simulink model "MLP_networks"  (Simulink 7.7)
settings: Solver=ode45  StartTime=0.0  StopTime=10.0  RelTol=1e-3
libraries: neural x1629
(part 39 of 39)

== system MLP_networks/net_loc_rod_8_9/Layer 2/LW{2,1} ==
  "ad{2,1}" : Inport  PortDimensions=25
      mask Display: e = 0.06;c1 = [120 230 180]/255;c2 = ([120 230 180]+0)/(256+128);c3 = ([120 230 180]+128)/(256+128);patch([0 1 1 0],[0 0 1 1],c1);patch([0 1 1 1-e 1-e 0+e],[0 0 1 1-e 0+e 0+e],c2);patch([0 0 1 1-e 0+e 0+e],[0 1 1 1-e 1-e 0+e],c3);plot([0 1 1 0 0],[0 0 1 1 0]);
  "IW{2,1}(1,:)'" : Constant  Value=[-0.45447080635271114;-0.31431087999466095;0.23643842966814058;-0.26838264066697265;0.62158079059535698;0.64630925965078334;0.21776904252102494;0.92838649448024702;0.73391848601792298;-0.68443553978244875;-0.058262504733950955;-0.71107335585701004;-0.54591324791636819;0.31074562654655796;-0.94685307026245902;0.26887324589974526;0.010705518827699401;0.3796394579843112;0.34327649941262317;-1.1437670216094;0.90053987028130467;-0.10901199864440488;-1.1073873884529284;-0.86410791260520914;-0.92204914739905952]
      mask Display: e = 0.06;c1 = [120 150 230]/255;c2 = ([120 150 230]+0)/383;c3 = ([120 150 230]+128)/383;patch([0 1 1 0],[0 0 1 1],c1);patch([0 1 1 1-e 1-e 0+e],[0 0 1 1-e 0+e 0+e],c2);patch([0 0 1 1-e 0+e 0+e],[0 1 1 1-e 1-e 0+e],c3);plot([0 1 1 0 0],[0 0 1 1 0]);disp('weights');
  "IW{2,1}(10,:)'" : Constant  Value=[0.16261320114205341;0.85057219130381734;0.55243127341530673;-0.88195117415749713;-0.30049390446276986;-1.014955763686713;-0.41393637036512715;-0.93954442090004908;-0.56215105670641552;0.52952072507725989;0.85440080646791894;-0.00250141878530565;-0.2902870234308268;0.77038178692241177;1.0193322993447076;-0.29348678456992017;-0.45281217341190522;-0.45486860238087545;1.084604474121075;0.56344685224125202;-0.6458534409188561;0.86989576896543919;-0.67894851658584343;-0.072787712075929586;-0.088449026765616598]
      mask Display: e = 0.06;c1 = [120 150 230]/255;c2 = ([120 150 230]+0)/383;c3 = ([120 150 230]+128)/383;patch([0 1 1 0],[0 0 1 1],c1);patch([0 1 1 1-e 1-e 0+e],[0 0 1 1-e 0+e 0+e],c2);patch([0 0 1 1-e 0+e 0+e],[0 1 1 1-e 1-e 0+e],c3);plot([0 1 1 0 0],[0 0 1 1 0]);disp('weights');
  "IW{2,1}(11,:)'" : Constant  Value=[0.51216797701577244;-0.61438892099831866;1.2332181859604123;-1.2152438498115505;0.52251736025113349;-0.13914170551847893;-0.89663294252450099;0.1071591841447891;0.64626961438857278;-0.31974975626390789;0.90425624594228193;0.23311810869026173;0.57809497930447595;-0.51759015720995505;0.65776609000005626;-0.056587943103239377;1.0934578461807081;0.20012077737366696;0.38928601290892856;-0.069925753988291706;-0.46833581265105323;-0.56124207265295978;-0.89459244639724333;-0.70694327274206104;0.41313009557411701]
      mask Display: e = 0.06;c1 = [120 150 230]/255;c2 = ([120 150 230]+0)/383;c3 = ([120 150 230]+128)/383;patch([0 1 1 0],[0 0 1 1],c1);patch([0 1 1 1-e 1-e 0+e],[0 0 1 1-e 0+e 0+e],c2);patch([0 0 1 1-e 0+e 0+e],[0 1 1 1-e 1-e 0+e],c3);plot([0 1 1 0 0],[0 0 1 1 0]);disp('weights');
  "IW{2,1}(12,:)'" : Constant  Value=[-1.0367153164928766;-0.2086773626137968;-0.80832015596878137;0.1947198621022756;0.49348641081723604;0.044812146591478745;0.93317961128790405;-0.84837718445793697;-0.36841126818182129;-1.1224562126356763;-1.3423580142895108;-0.84409074802752404;-0.91276151182855159;-0.12584803107768913;-0.3402152433083459;-0.44504069889487502;-0.13012390121533071;0.46056376582825703;0.99075176834323464;0.095867520968736894;-0.58086488598308128;0.34331851844642508;1.0804134362946722;0.57636843085678846;0.0068501557111167151]
      mask Display: e = 0.06;c1 = [120 150 230]/255;c2 = ([120 150 230]+0)/383;c3 = ([120 150 230]+128)/383;patch([0 1 1 0],[0 0 1 1],c1);patch([0 1 1 1-e 1-e 0+e],[0 0 1 1-e 0+e 0+e],c2);patch([0 0 1 1-e 0+e 0+e],[0 1 1 1-e 1-e 0+e],c3);plot([0 1 1 0 0],[0 0 1 1 0]);disp('weights');
  "IW{2,1}(13,:)'" : Constant  Value=[-0.7243727430640643;-0.75325987047203258;0.32916868557887041;-0.87046233057132527;-0.40505034549515351;-0.73606709995248509;-0.57117708847133197;-0.028661557321403193;-0.12907256376571835;-0.70882230384049871;0.31678226521368041;-0.10082364388092978;0.6564749890771453;-0.049738012916444661;0.83422659334940041;-1.1296704058541949;0.94089271777742445;0.15949922140755984;-0.10705922974869457;0.87697187766797047;-1.0866913744390712;-0.71353658871453851;-0.31873702515843627;-0.252881252085425;-1.0189008728429951]
      mask Display: e = 0.06;c1 = [120 150 230]/255;c2 = ([120 150 230]+0)/383;c3 = ([120 150 230]+128)/383;patch([0 1 1 0],[0 0 1 1],c1);patch([0 1 1 1-e 1-e 0+e],[0 0 1 1-e 0+e 0+e],c2);patch([0 0 1 1-e 0+e 0+e],[0 1 1 1-e 1-e 0+e],c3);plot([0 1 1 0 0],[0 0 1 1 0]);disp('weights');
  "IW{2,1}(14,:)'" : Constant  Value=[0.53371665285306602;-0.76095279927957649;-0.094308089491326283;0.80974430444344658;-1.0601529091744661;-0.57891757482366835;0.032455299426623785;-0.37525233439382483;-0.8579469021295838;0.83494699788668525;0.049205853924271216;-0.77709270533384189;0.19868335805748968;-0.88504930806369408;-0.095340804143279015;0.52800234434791515;-0.43233621624610419;-0.64289579789318352;0.75364398055159043;0.77792715087691144;0.63464043036909801;-0.21444243504652935;0.52064758843423997;-0.90369622137036576;-0.93600425626526274]
      mask Display: e = 0.06;c1 = [120 150 230]/255;c2 = ([120 150 230]+0)/383;c3 = ([120 150 230]+128)/383;patch([0 1 1 0],[0 0 1 1],c1);patch([0 1 1 1-e 1-e 0+e],[0 0 1 1-e 0+e 0+e],c2);patch([0 0 1 1-e 0+e 0+e],[0 1 1 1-e 1-e 0+e],c3);plot([0 1 1 0 0],[0 0 1 1 0]);disp('weights');
  "IW{2,1}(15,:)'" : Constant  Value=[0.37541716291702742;-0.21193619710435674;-0.94576323987022948;0.34691220420858604;-0.38907419761502582;0.84729396197252627;0.61247771158965003;1.0019605765670976;-0.045197648782573069;-1.1799168746424504;0.84852837950369564;-0.81099574040787803;0.1941658430896363;-0.010229454310141418;0.44591624310136047;-0.38010130538266051;-0.75205589528395445;0.60044481822345563;0.82055369407816969;0.053523240861982138;1.2391033690142557;-0.54989802212004923;-0.14511814137346626;-0.33145647268207051;0.56500446191282006]
      mask Display: e = 0.06;c1 = [120 150 230]/255;c2 = ([120 150 230]+0)/383;c3 = ([120 150 230]+128)/383;patch([0 1 1 0],[0 0 1 1],c1);patch([0 1 1 1-e 1-e 0+e],[0 0 1 1-e 0+e 0+e],c2);patch([0 0 1 1-e 0+e 0+e],[0 1 1 1-e 1-e 0+e],c3);plot([0 1 1 0 0],[0 0 1 1 0]);disp('weights');
  "IW{2,1}(16,:)'" : Constant  Value=[-1.0394652666780868;0.15085289490948153;0.44339428350864968;-0.77309686754184659;-0.33808340538731163;-1.1935669085568268;-0.63097259795222405;0.299249348653851;0.92160773792947315;-1.0044893892944822;0.40875287808051819;-0.12022115639313204;-0.4889679626946678;1.0578373529209588;0.6070540991902259;0.9876432388180314;0.32942173306276984;0.08451986358521997;-0.1855524467079297;0.70927078909658214;0.77583003077482993;-0.087847247331581058;0.58774596387649525;-0.62544316719270998;-0.35284088943191494]
      mask Display: e = 0.06;c1 = [120 150 230]/255;c2 = ([120 150 230]+0)/383;c3 = ([120 150 230]+128)/383;patch([0 1 1 0],[0 0 1 1],c1);patch([0 1 1 1-e 1-e 0+e],[0 0 1 1-e 0+e 0+e],c2);patch([0 0 1 1-e 0+e 0+e],[0 1 1 1-e 1-e 0+e],c3);plot([0 1 1 0 0],[0 0 1 1 0]);disp('weights');
  "IW{2,1}(17,:)'" : Constant  Value=[0.34126724354609184;0.73618068075490573;0.61771615039297245;-0.75619007627092016;0.098089840878866116;-0.966566899104913;0.5073556368631954;1.027292936105652;0.21560095819971478;-0.2639067977294588;-0.710128333782023;-0.35468195912204459;0.62972345593633328;0.088918966245724623;-0.57676352850483459;0.59235109654670703;0.62310731853968448;1.0120009144022506;0.28344383729740075;-0.67135974215603889;0.53291075314000347;0.92992562657934774;0.045942961126403739;-0.97360891231881208;-0.8952773597675806]
      mask Display: e = 0.06;c1 = [120 150 230]/255;c2 = ([120 150 230]+0)/383;c3 = ([120 150 230]+128)/383;patch([0 1 1 0],[0 0 1 1],c1);patch([0 1 1 1-e 1-e 0+e],[0 0 1 1-e 0+e 0+e],c2);patch([0 0 1 1-e 0+e 0+e],[0 1 1 1-e 1-e 0+e],c3);plot([0 1 1 0 0],[0 0 1 1 0]);disp('weights');
  "IW{2,1}(18,:)'" : Constant  Value=[-0.098397319648461698;-1.1310897911939402;0.20417535507397502;-0.7539013471598266;0.68442491292076157;0.25093656866891895;-1.1397774937477676;0.12159248155228496;0.7780135310512547;0.035538843403749382;-0.91235298915348495;-1.0000341549927907;0.79208580035862641;0.00074876713405867118;-0.31150935626008885;-0.96556344356727131;-0.4361193934911502;0.1376261764682912;0.59882639597992626;-0.42398383503226761;1.1604296296421897;-0.21284418619408138;0.34961610435553286;0.084401125103079372;-0.72242990170213894]
      mask Display: e = 0.06;c1 = [120 150 230]/255;c2 = ([120 150 230]+0)/383;c3 = ([120 150 230]+128)/383;patch([0 1 1 0],[0 0 1 1],c1);patch([0 1 1 1-e 1-e 0+e],[0 0 1 1-e 0+e 0+e],c2);patch([0 0 1 1-e 0+e 0+e],[0 1 1 1-e 1-e 0+e],c3);plot([0 1 1 0 0],[0 0 1 1 0]);disp('weights');
  "IW{2,1}(19,:)'" : Constant  Value=[0.78773378785982129;-0.48036277769725011;-0.47045729207981185;-1.0285380769624823;0.57946471346881834;-1.0274103528129928;-0.48201049424572456;0.33639731381638377;0.83791439406269541;-0.74451317574282194;-0.51790206635491542;0.25105315003569045;0.48285725406315255;0.81142022830880567;-0.93247588992234043;-0.62647816753072572;0.15040280733987643;0.65792099584298835;0.37927369980568609;-0.81003399537479481;-0.62849242597305155;0.068466355370222956;-0.30458643155508885;0.08181346905433419;-0.87104728264235998]
      mask Display: e = 0.06;c1 = [120 150 230]/255;c2 = ([120 150 230]+0)/383;c3 = ([120 150 230]+128)/383;patch([0 1 1 0],[0 0 1 1],c1);patch([0 1 1 1-e 1-e 0+e],[0 0 1 1-e 0+e 0+e],c2);patch([0 0 1 1-e 0+e 0+e],[0 1 1 1-e 1-e 0+e],c3);plot([0 1 1 0 0],[0 0 1 1 0]);disp('weights');
  "IW{2,1}(2,:)'" : Constant  Value=[0.96230663942317574;-0.44935662887228023;-0.56623021211938263;-0.98970111008255923;-0.17258463946061253;-0.86731106367562238;0.74381718631924409;0.6694547609833591;0.75417674683607538;-1.0130175782751791;0.99952362222759994;0.37793136884111361;-0.5244440690711103;-0.34430315584704518;-0.78883180270087583;0.74499763515124462;0.34936053745594026;-0.28074185014234565;-0.59199610119552726;0.28196716663522736;0.95011394088102452;-0.69131758403450982;-0.05622148048795448;-0.85996969469457929;0.28393870377919894]
      mask Display: e = 0.06;c1 = [120 150 230]/255;c2 = ([120 150 230]+0)/383;c3 = ([120 150 230]+128)/383;patch([0 1 1 0],[0 0 1 1],c1);patch([0 1 1 1-e 1-e 0+e],[0 0 1 1-e 0+e 0+e],c2);patch([0 0 1 1-e 0+e 0+e],[0 1 1 1-e 1-e 0+e],c3);plot([0 1 1 0 0],[0 0 1 1 0]);disp('weights');
  "IW{2,1}(20,:)'" : Constant  Value=[0.86417986057223173;-0.71409214147296729;0.87649163618636761;-0.26966100345125088;0.22235648369379468;0.58221344515541951;0.49784067504208446;0.97207961406944532;0.9071543515886572;0.68777222135818183;-0.042949087236494599;0.59168218732534095;-0.12077111467202464;0.79259172488769247;-0.45576896748524726;-0.50437719394637759;-0.70249062368748016;0.89245706256996071;0.88961506239928179;0.72849965232042246;-0.026521615511835725;0.079500787307071025;-0.43713934870209875;-0.80163782346974666;-0.83869567670330147]
      mask Display: e = 0.06;c1 = [120 150 230]/255;c2 = ([120 150 230]+0)/383;c3 = ([120 150 230]+128)/383;patch([0 1 1 0],[0 0 1 1],c1);patch([0 1 1 1-e 1-e 0+e],[0 0 1 1-e 0+e 0+e],c2);patch([0 0 1 1-e 0+e 0+e],[0 1 1 1-e 1-e 0+e],c3);plot([0 1 1 0 0],[0 0 1 1 0]);disp('weights');
  "IW{2,1}(21,:)'" : Constant  Value=[0.1911532386158688;0.1621449493425382;-0.93637196968629799;-0.26400809382302576;0.54569865597064104;0.88748772662652009;0.50077218719541849;0.67412697249317532;0.40883495027129241;-0.092833189717247674;-0.74794325847843501;-0.60048439500264339;0.40310127003620538;-0.28964783835670249;-0.94317412015928992;0.85095667464863523;-0.17069104715442765;0.58499249929003749;-1.0048085585643964;0.23236160394851982;-0.48000714163089853;-1.000876063264845;0.99191080162000533;0.80503319313583599;-0.51157270112970599]
      mask Display: e = 0.06;c1 = [120 150 230]/255;c2 = ([120 150 230]+0)/383;c3 = ([120 150 230]+128)/383;patch([0 1 1 0],[0 0 1 1],c1);patch([0 1 1 1-e 1-e 0+e],[0 0 1 1-e 0+e 0+e],c2);patch([0 0 1 1-e 0+e 0+e],[0 1 1 1-e 1-e 0+e],c3);plot([0 1 1 0 0],[0 0 1 1 0]);disp('weights');
  "IW{2,1}(22,:)'" : Constant  Value=[0.9320611787902402;0.28364314918527139;-0.20093614072570032;-0.3751052916383622;-0.52578913527537752;0.70237214101441625;-1.0319590808387713;-0.85558263819382308;0.88270969846196012;-0.46751281861565375;-0.91417776486314584;0.31547930902410298;0.81163899116420279;-0.15828942492757292;-0.24707285170931548;-0.39170449380734118;-0.88386960061365805;1.1541453664581989;0.78038688405888279;0.5306796455286874;0.34440910112714629;-0.33799086462182248;0.8850373797599308;-0.63028138227995167;0.17673160463486462]
      mask Display: e = 0.06;c1 = [120 150 230]/255;c2 = ([120 150 230]+0)/383;c3 = ([120 150 230]+128)/383;patch([0 1 1 0],[0 0 1 1],c1);patch([0 1 1 1-e 1-e 0+e],[0 0 1 1-e 0+e 0+e],c2);patch([0 0 1 1-e 0+e 0+e],[0 1 1 1-e 1-e 0+e],c3);plot([0 1 1 0 0],[0 0 1 1 0]);disp('weights');
  "IW{2,1}(23,:)'" : Constant  Value=[-0.82185203974927235;0.92891702155408973;-0.37877676349477202;-0.62190517768300357;0.32818732774692172;0.0038303412033409774;-0.14571980217775737;0.80249850052066751;-0.63021858125598862;0.78492448828022865;-0.94038973664783887;0.71945342383225364;-0.93285472625417609;-0.32614841235081482;0.73697057015097023;-0.38846684548949634;0.88920720011482535;0.20290850509137778;-0.84560863661300678;-0.16868606751307699;-0.84819165523872442;-0.40115615282001765;-0.65920959088980569;0.72810794552070213;-0.25217760313611665]
      mask Display: e = 0.06;c1 = [120 150 230]/255;c2 = ([120 150 230]+0)/383;c3 = ([120 150 230]+128)/383;patch([0 1 1 0],[0 0 1 1],c1);patch([0 1 1 1-e 1-e 0+e],[0 0 1 1-e 0+e 0+e],c2);patch([0 0 1 1-e 0+e 0+e],[0 1 1 1-e 1-e 0+e],c3);plot([0 1 1 0 0],[0 0 1 1 0]);disp('weights');
  "IW{2,1}(24,:)'" : Constant  Value=[0.30582931147396802;-0.036178013157462559;-0.55531656899262816;0.76280973892360027;-0.03762136036114589;-0.76339575584342301;0.99723793513686021;-0.48053176437438622;0.7936960673034823;-0.47389009352160244;-0.12021842780939135;-1.0176735468094926;1.0051963883138231;0.53389548534064435;0.62406304753365782;-0.45167165089064937;-0.18484523206284098;-0.88667933177244607;0.59183228168738489;-0.71299173383454761;0.59431335267309748;-0.83985050387188986;0.59717562904826715;0.75949420856795158;0.39693109681614497]
      mask Display: e = 0.06;c1 = [120 150 230]/255;c2 = ([120 150 230]+0)/383;c3 = ([120 150 230]+128)/383;patch([0 1 1 0],[0 0 1 1],c1);patch([0 1 1 1-e 1-e 0+e],[0 0 1 1-e 0+e 0+e],c2);patch([0 0 1 1-e 0+e 0+e],[0 1 1 1-e 1-e 0+e],c3);plot([0 1 1 0 0],[0 0 1 1 0]);disp('weights');
  "IW{2,1}(25,:)'" : Constant  Value=[-1.0684009758474187;1.1722115613612545;-0.57111187175963052;-0.8878679369744843;1.1295127330090828;0.44904490314857132;0.14031476727547645;0.08735425437740639;-0.34565747025485005;-0.72178721361568943;0.59197326673989126;-0.42068869129676106;-0.82095323234120809;-0.82414047258516032;0.056752643726297583;-0.0579096547071552;0.271312447793641;0.89147339407483417;0.17874804668826502;-0.10936602263727534;0.3520689038399139;-0.76695586884888844;-0.43345975693307037;0.88579403742493612;0.47182323470607712]
      mask Display: e = 0.06;c1 = [120 150 230]/255;c2 = ([120 150 230]+0)/383;c3 = ([120 150 230]+128)/383;patch([0 1 1 0],[0 0 1 1],c1);patch([0 1 1 1-e 1-e 0+e],[0 0 1 1-e 0+e 0+e],c2);patch([0 0 1 1-e 0+e 0+e],[0 1 1 1-e 1-e 0+e],c3);plot([0 1 1 0 0],[0 0 1 1 0]);disp('weights');
  "IW{2,1}(26,:)'" : Constant  Value=[0.77450591200359475;0.91270531388688547;0.83574788691334789;-0.34502986728419421;-0.55790971192747163;-0.72070283837337334;0.20504475257688248;-0.83640939284270199;0.64277075785744209;-0.57192213445216011;0.32327000181573323;-0.68416799747796198;-0.90528107143746939;-0.10217138652846579;0.73971597769657271;0.89218725128765564;0.29840745150663905;-0.5450647450867212;-0.73235030444179139;-0.58115961231792035;0.63460766784378642;0.40333367981231855;-0.89475280670748758;0.65293566293097571;0.12099389597776294]
      mask Display: e = 0.06;c1 = [120 150 230]/255;c2 = ([120 150 230]+0)/383;c3 = ([120 150 230]+128)/383;patch([0 1 1 0],[0 0 1 1],c1);patch([0 1 1 1-e 1-e 0+e],[0 0 1 1-e 0+e 0+e],c2);patch([0 0 1 1-e 0+e 0+e],[0 1 1 1-e 1-e 0+e],c3);plot([0 1 1 0 0],[0 0 1 1 0]);disp('weights');
  "IW{2,1}(27,:)'" : Constant  Value=[0.61217593788432589;1.0105744665838057;0.10860586955594799;0.94251107889473051;-0.88010468086265536;1.0106862859418371;0.97539560690599569;0.50827419220215719;0.59801040058874899;-0.039371834639818012;0.42615970864737573;0.40800828356563923;0.5757827372943547;0.85016099941120338;0.89746531145472463;0.080547975206119823;0.090172289218227619;-0.87795208623074783;0.69526781873484145;-0.45630044385637419;-0.17710867995277463;0.76421683404438578;-0.41404996922286047;-0.32332715019168495;-0.36597634722835087]
      mask Display: e = 0.06;c1 = [120 150 230]/255;c2 = ([120 150 230]+0)/383;c3 = ([120 150 230]+128)/383;patch([0 1 1 0],[0 0 1 1],c1);patch([0 1 1 1-e 1-e 0+e],[0 0 1 1-e 0+e 0+e],c2);patch([0 0 1 1-e 0+e 0+e],[0 1 1 1-e 1-e 0+e],c3);plot([0 1 1 0 0],[0 0 1 1 0]);disp('weights');
  "IW{2,1}(28,:)'" : Constant  Value=[-0.92362832193853739;0.29233412368150907;-0.28036118684992595;-0.52775115853329257;1.1089509079989204;0.17905600152632489;0.46663393694438871;-0.37191504490185906;-0.17999421651757258;0.058306317753163014;-1.0140410146243994;-0.11183420954904957;0.98413115720863986;0.16517689889845533;0.88854308219033906;-1.0667065996248886;0.60226014665316829;-0.96893529625524433;-0.5008750006416941;0.022413819844856471;-0.62628687438953801;0.42127137893488054;0.15159245687022385;1.0789682742542015;0.56723459454054859]
      mask Display: e = 0.06;c1 = [120 150 230]/255;c2 = ([120 150 230]+0)/383;c3 = ([120 150 230]+128)/383;patch([0 1 1 0],[0 0 1 1],c1);patch([0 1 1 1-e 1-e 0+e],[0 0 1 1-e 0+e 0+e],c2);patch([0 0 1 1-e 0+e 0+e],[0 1 1 1-e 1-e 0+e],c3);plot([0 1 1 0 0],[0 0 1 1 0]);disp('weights');
  "IW{2,1}(29,:)'" : Constant  Value=[-0.75071122167525839;-0.16377370234095223;1.0432309786139491;-0.9419284667685428;0.76379982457742834;0.43959955342497242;-0.76278982989123456;0.10257817545510309;0.74004434461333557;0.83753673819670804;0.13167611675610816;0.76014534213608953;-0.66457009872673756;0.36592785804355776;-0.6120363225355574;-0.488276829481398;-0.6618208484555782;-0.11194073805334005;0.22043830882817622;-0.40349829775212342;0.47209337717495281;-0.87514000467748676;-0.74737020827019207;-0.96943693375218565;0.64256521052270565]
      mask Display: e = 0.06;c1 = [120 150 230]/255;c2 = ([120 150 230]+0)/383;c3 = ([120 150 230]+128)/383;patch([0 1 1 0],[0 0 1 1],c1);patch([0 1 1 1-e 1-e 0+e],[0 0 1 1-e 0+e 0+e],c2);patch([0 0 1 1-e 0+e 0+e],[0 1 1 1-e 1-e 0+e],c3);plot([0 1 1 0 0],[0 0 1 1 0]);disp('weights');
  "IW{2,1}(3,:)'" : Constant  Value=[-0.72661874690638639;0.98304485670167907;-0.39280364502085141;0.30668407085875982;-0.230114863701743;0.43303809144138394;0.7277239726221405;0.99977015994841312;0.87853696172551077;0.1970889781751029;-0.97320525276089309;0.56460947642782677;0.32677707421560953;-0.32048198505949954;0.50614504721549824;-0.45383421909495375;0.92994931318815421;-0.39720128292223061;0.92109540405251633;-0.71483440373770279;0.85524274992117122;-0.069813992173348174;-0.5834831065067082;0.81005318020036188;0.33671550153450908]
      mask Display: e = 0.06;c1 = [120 150 230]/255;c2 = ([120 150 230]+0)/383;c3 = ([120 150 230]+128)/383;patch([0 1 1 0],[0 0 1 1],c1);patch([0 1 1 1-e 1-e 0+e],[0 0 1 1-e 0+e 0+e],c2);patch([0 0 1 1-e 0+e 0+e],[0 1 1 1-e 1-e 0+e],c3);plot([0 1 1 0 0],[0 0 1 1 0]);disp('weights');
  "IW{2,1}(30,:)'" : Constant  Value=[0.9520365997944269;0.5784099977345214;0.74134421413668339;-0.06363803828697058;-1.0124114735802598;-0.093182754887791014;-0.20269235928731327;-0.094131170798026784;0.80239368351042095;0.27621364652589353;-0.39945726685966931;0.38509994188586416;0.76957868255844897;-0.55737306059620473;0.88795019251236396;1.2044289516558007;0.13452228364405522;0.51460777295093929;0.3092540981712541;-0.68222047984635237;0.01906913268519532;-0.37617379142855234;0.93628982587397003;-1.0441754001006984;0.068380270421470518]
      mask Display: e = 0.06;c1 = [120 150 230]/255;c2 = ([120 150 230]+0)/383;c3 = ([120 150 230]+128)/383;patch([0 1 1 0],[0 0 1 1],c1);patch([0 1 1 1-e 1-e 0+e],[0 0 1 1-e 0+e 0+e],c2);patch([0 0 1 1-e 0+e 0+e],[0 1 1 1-e 1-e 0+e],c3);plot([0 1 1 0 0],[0 0 1 1 0]);disp('weights');
  "IW{2,1}(31,:)'" : Constant  Value=[0.15567714868126017;-0.072085627004655969;-0.050397630838470736;0.95833156808844622;-0.1879410696794612;-0.59649025386386878;0.84553357656875139;0.61551922306369911;-0.9713825097799843;0.4979667076348453;0.26631163648564493;-0.17892940121863304;-0.051055201034569529;-1.1033606312967341;-0.18636221888045618;1.2140195934896645;-0.43500698384749537;-0.51998517385757448;-1.1353997625882177;0.85700759160672535;0.47407089976182043;-0.51827476400697037;0.06559682343247443;-0.911672680644522;-0.15377455532303921]
      mask Display: e = 0.06;c1 = [120 150 230]/255;c2 = ([120 150 230]+0)/383;c3 = ([120 150 230]+128)/383;patch([0 1 1 0],[0 0 1 1],c1);patch([0 1 1 1-e 1-e 0+e],[0 0 1 1-e 0+e 0+e],c2);patch([0 0 1 1-e 0+e 0+e],[0 1 1 1-e 1-e 0+e],c3);plot([0 1 1 0 0],[0 0 1 1 0]);disp('weights');
  "IW{2,1}(32,:)'" : Constant  Value=[0.82909455037823787;0.99714319599564616;1.1139332023334763;0.54654892769062013;0.52131269431691585;-0.80449944267326734;0.55664826096035924;-1.002741723350306;-0.01985018005497385;-0.67254734982516517;-0.93662079473490822;-0.03014214992894999;1.0464148662521608;0.15910202671912124;1.2862964972491364;0.45764157957773155;0.71356320912522109;-0.42510632495263323;-0.69440295242741623;-0.0045543062036582822;0.035464232309733092;-0.19904714832607096;0.1444002491346317;0.040868735796712262;0.083526646292963455]
      mask Display: e = 0.06;c1 = [120 150 230]/255;c2 = ([120 150 230]+0)/383;c3 = ([120 150 230]+128)/383;patch([0 1 1 0],[0 0 1 1],c1);patch([0 1 1 1-e 1-e 0+e],[0 0 1 1-e 0+e 0+e],c2);patch([0 0 1 1-e 0+e 0+e],[0 1 1 1-e 1-e 0+e],c3);plot([0 1 1 0 0],[0 0 1 1 0]);disp('weights');
  "IW{2,1}(33,:)'" : Constant  Value=[0.036631572386991482;-0.4859312403210907;0.47210982987621547;0.89311539401184092;0.62724039374736873;-0.75762622064522089;-0.22116005207619702;-1.0000476620174505;0.88242383389663503;0.87406908733565825;0.27178801741200337;-0.85961354623926522;0.80446421087919417;0.94536513407364309;0.67862529152930817;-0.11239854292815231;0.48071669928340838;-0.21685603275548129;-0.018082263103240091;-1.0018384755236334;-0.74941988688188865;0.14514850868224274;0.19341587119424772;-0.95315483233896936;0.087088605244087264]
      mask Display: e = 0.06;c1 = [120 150 230]/255;c2 = ([120 150 230]+0)/383;c3 = ([120 150 230]+128)/383;patch([0 1 1 0],[0 0 1 1],c1);patch([0 1 1 1-e 1-e 0+e],[0 0 1 1-e 0+e 0+e],c2);patch([0 0 1 1-e 0+e 0+e],[0 1 1 1-e 1-e 0+e],c3);plot([0 1 1 0 0],[0 0 1 1 0]);disp('weights');
  "IW{2,1}(34,:)'" : Constant  Value=[0.53373781853001401;1.0854542172297528;-0.050268462275507235;0.18814361980720323;-0.19858976628212019;0.95097137761216377;-1.0046101954080138;-0.16748350752219901;-0.072886125187907491;-0.95017139866892542;-0.7534524616942313;-1.0120494484012044;-0.30821221046317987;0.3623711234025066;-0.032567929132316251;-1.1176982715758284;0.19097961349793782;0.37497120131263378;0.69756716041654054;0.97114030711281907;-0.99072273810272415;0.32529142645115866;0.5459282808151813;-0.46238529402502659;0.31491921013096502]
      mask Display: e = 0.06;c1 = [120 150 230]/255;c2 = ([120 150 230]+0)/383;c3 = ([120 150 230]+128)/383;patch([0 1 1 0],[0 0 1 1],c1);patch([0 1 1 1-e 1-e 0+e],[0 0 1 1-e 0+e 0+e],c2);patch([0 0 1 1-e 0+e 0+e],[0 1 1 1-e 1-e 0+e],c3);plot([0 1 1 0 0],[0 0 1 1 0]);disp('weights');
  "IW{2,1}(35,:)'" : Constant  Value=[0.51979428844107578;0.80936660991970011;0.89434175320810017;0.22804712757419968;-0.39797463477756434;-0.16323079404302634;-0.28184633595783565;-0.80960057310033162;-0.91452441576709198;-0.70296872148801859;0.34996440277301383;0.60428302086858032;-0.33764774632615158;-0.9516367577091448;0.17289559134218208;1.0099555310096149;0.65922170646939704;-0.90277879989919618;0.61983937615839846;-0.93840826454856285;-0.50370480019087227;-0.47833541448699218;-0.85582425731092604;0.37359779335281229;-0.60469184067102733]
      mask Display: e = 0.06;c1 = [120 150 230]/255;c2 = ([120 150 230]+0)/383;c3 = ([120 150 230]+128)/383;patch([0 1 1 0],[0 0 1 1],c1);patch([0 1 1 1-e 1-e 0+e],[0 0 1 1-e 0+e 0+e],c2);patch([0 0 1 1-e 0+e 0+e],[0 1 1 1-e 1-e 0+e],c3);plot([0 1 1 0 0],[0 0 1 1 0]);disp('weights');
  "IW{2,1}(36,:)'" : Constant  Value=[-0.23384974203236852;-0.54113992244807474;1.1016650872942653;1.1867094141570538;-0.18259887724139948;-0.61650306840294833;-1.0579748981135972;-0.86695949316505472;0.34258323344695207;0.25134154100917466;0.49668598978421058;1.0874547853160808;0.33877522986499109;0.07278981615384239;-0.93246428697756634;-0.49415699510248245;-0.61347936617450993;0.96312184078209462;-0.31995152917786074;-0.49914549720953977;0.26822355945592924;-0.66445453280374978;0.065126988778028916;-0.74467649600230734;0.31341549290898102]
      mask Display: e = 0.06;c1 = [120 150 230]/255;c2 = ([120 150 230]+0)/383;c3 = ([120 150 230]+128)/383;patch([0 1 1 0],[0 0 1 1],c1);patch([0 1 1 1-e 1-e 0+e],[0 0 1 1-e 0+e 0+e],c2);patch([0 0 1 1-e 0+e 0+e],[0 1 1 1-e 1-e 0+e],c3);plot([0 1 1 0 0],[0 0 1 1 0]);disp('weights');
  "IW{2,1}(37,:)'" : Constant  Value=[0.62394894755522512;-0.72463106030111668;-0.28915310904051367;0.38031615254904;0.96336050725290678;0.94026979907725095;0.45200410654678858;0.77127112338602177;-0.42381660866722354;-1.0203299574836318;0.055877914679506882;-0.46593533880670451;0.91323202709270723;-0.86505688276390513;0.021478310200374332;0.9544367752917674;-0.70347566787313309;-0.54726505052392349;-0.56606452403588858;0.78215767993104612;0.40928629022026891;0.078962355906479584;-0.84847545453080819;0.16386319596577098;-0.48167518437484919]
      mask Display: e = 0.06;c1 = [120 150 230]/255;c2 = ([120 150 230]+0)/383;c3 = ([120 150 230]+128)/383;patch([0 1 1 0],[0 0 1 1],c1);patch([0 1 1 1-e 1-e 0+e],[0 0 1 1-e 0+e 0+e],c2);patch([0 0 1 1-e 0+e 0+e],[0 1 1 1-e 1-e 0+e],c3);plot([0 1 1 0 0],[0 0 1 1 0]);disp('weights');
  "IW{2,1}(38,:)'" : Constant  Value=[-0.82263192954369435;0.37012724951292331;0.74972080760741266;1.0351005528830399;0.56512505853040529;-0.81539680330377129;0.39072051088000676;-0.29041608151021198;-0.0087149107531334213;0.74173699894930678;0.11484230430867111;0.87839370487535939;0.2494334766034727;0.11682233387751935;0.69415268384814743;-0.04027180420643884;-0.11770698203286697;-0.1421206021269576;0.67417577094500547;-0.75587535966966957;-1.1957762438779307;0.89939892311584302;-0.77485709288092064;0.10804837880923522;1.1712256256702318]
      mask Display: e = 0.06;c1 = [120 150 230]/255;c2 = ([120 150 230]+0)/383;c3 = ([120 150 230]+128)/383;patch([0 1 1 0],[0 0 1 1],c1);patch([0 1 1 1-e 1-e 0+e],[0 0 1 1-e 0+e 0+e],c2);patch([0 0 1 1-e 0+e 0+e],[0 1 1 1-e 1-e 0+e],c3);plot([0 1 1 0 0],[0 0 1 1 0]);disp('weights');
  "IW{2,1}(39,:)'" : Constant  Value=[-0.087941008322375919;-1.2617558070192225;0.81267471888099152;-0.095310299855226308;-0.14430690024522641;-0.59215209219935194;-0.24621944251458036;1.0141764718422999;-0.72126979904741317;-0.24786972627093884;-0.85079063426578938;-0.2060494957307637;0.17468343830161173;-0.20772011445927371;0.83117698885287106;-0.8259244632319398;-0.72584811323123788;-0.50446335809251608;0.30702358162880289;-0.22927699911977933;0.7303610645550993;-0.67473178861566885;0.565406694916473;0.0085444645835071244;1.2613327692520118]
      mask Display: e = 0.06;c1 = [120 150 230]/255;c2 = ([120 150 230]+0)/383;c3 = ([120 150 230]+128)/383;patch([0 1 1 0],[0 0 1 1],c1);patch([0 1 1 1-e 1-e 0+e],[0 0 1 1-e 0+e 0+e],c2);patch([0 0 1 1-e 0+e 0+e],[0 1 1 1-e 1-e 0+e],c3);plot([0 1 1 0 0],[0 0 1 1 0]);disp('weights');
  "IW{2,1}(4,:)'" : Constant  Value=[-0.91763924018682308;-0.14482416183886465;-0.81975295697163553;0.50338071021686293;1.1036741771908423;0.31005456238123802;0.86665074311709989;0.30585124448433609;0.051290156212662578;-0.6974987566200439;0.18478498207816629;0.47363312320663153;-0.073589393868213546;-1.045358662826845;0.82981806326454777;0.95650149909522542;-0.37939447955152711;0.43646379385359629;0.076893257963874376;0.89801851174081115;1.0491188749862304;0.36373872441237598;0.37760536648727727;-0.47948700442506348;0.70507282134646909]
      mask Display: e = 0.06;c1 = [120 150 230]/255;c2 = ([120 150 230]+0)/383;c3 = ([120 150 230]+128)/383;patch([0 1 1 0],[0 0 1 1],c1);patch([0 1 1 1-e 1-e 0+e],[0 0 1 1-e 0+e 0+e],c2);patch([0 0 1 1-e 0+e 0+e],[0 1 1 1-e 1-e 0+e],c3);plot([0 1 1 0 0],[0 0 1 1 0]);disp('weights');
  "IW{2,1}(40,:)'" : Constant  Value=[0.10117395120403073;0.24715881593069883;0.83728045669710482;-0.18671601343198624;0.069509096529898423;-0.19742449946957311;0.83344649776616908;1.3106956705379531;-0.2462286395319955;-0.90486362677857146;0.54701955067878771;0.89670157241501358;0.35229560876483135;0.66802678717329667;0.063332974454404695;-0.46645975844027782;1.3814570160061039;-0.33411412115441702;-0.42341112280074589;-0.62588934616862224;-1.2228788212487895;-0.44646354140142547;0.23884228407282401;-0.9311058974493388;0.78530320127861797]
      mask Display: e = 0.06;c1 = [120 150 230]/255;c2 = ([120 150 230]+0)/383;c3 = ([120 150 230]+128)/383;patch([0 1 1 0],[0 0 1 1],c1);patch([0 1 1 1-e 1-e 0+e],[0 0 1 1-e 0+e 0+e],c2);patch([0 0 1 1-e 0+e 0+e],[0 1 1 1-e 1-e 0+e],c3);plot([0 1 1 0 0],[0 0 1 1 0]);disp('weights');
  "IW{2,1}(5,:)'" : Constant  Value=[1.0939965012744106;-0.66742083860121626;0.44176116557230544;0.19488103679144;-0.41864394361289581;-0.97783478160897297;-0.24004993526630705;-0.71760852479943238;0.65681332424103389;-0.21988704460819664;-0.5813359133985625;-0.34065285262784456;0.9033686873923521;-0.62892988549260465;0.88227040548382951;-0.98957493871181734;-0.18279002704064404;0.81324318493551628;-0.5523906417857144;0.64071395311200929;-0.44341231540924431;-0.70364701527976248;-0.55889331586038327;0.57611249338715798;-0.80142859703937419]
      mask Display: e = 0.06;c1 = [120 150 230]/255;c2 = ([120 150 230]+0)/383;c3 = ([120 150 230]+128)/383;patch([0 1 1 0],[0 0 1 1],c1);patch([0 1 1 1-e 1-e 0+e],[0 0 1 1-e 0+e 0+e],c2);patch([0 0 1 1-e 0+e 0+e],[0 1 1 1-e 1-e 0+e],c3);plot([0 1 1 0 0],[0 0 1 1 0]);disp('weights');
  "IW{2,1}(6,:)'" : Constant  Value=[0.52672972175919663;-0.54234069679748398;0.26229992785495393;-0.43950033724518695;-0.47671006602958749;-0.4084766690695722;-0.36069666513241849;0.96896850921895872;1.0365754228866313;0.016908975229810146;-0.48417792757850503;0.78272104705523271;-0.053406657320566486;0.41691219365676491;-0.50300491903087408;-1.2337188253843483;0.94909946627070729;-0.44246513377777069;-0.66330401220892377;-0.0034619098097734263;0.5949373079918362;0.48162040059480948;1.0523240380352006;0.89633573238191411;-0.36727415959127846]
      mask Display: e = 0.06;c1 = [120 150 230]/255;c2 = ([120 150 230]+0)/383;c3 = ([120 150 230]+128)/383;patch([0 1 1 0],[0 0 1 1],c1);patch([0 1 1 1-e 1-e 0+e],[0 0 1 1-e 0+e 0+e],c2);patch([0 0 1 1-e 0+e 0+e],[0 1 1 1-e 1-e 0+e],c3);plot([0 1 1 0 0],[0 0 1 1 0]);disp('weights');
  "IW{2,1}(7,:)'" : Constant  Value=[-0.92097304747775321;0.77184685775303008;0.59861696352770177;-0.90969894618776748;-0.2977289827858382;-0.42125420563932353;-0.30353431243711138;-0.79478270986220512;0.37036552308585063;0.96031032402227756;-0.5691407889005915;0.15789912485565882;0.081464386526960822;0.73206086220180977;-0.70793592161055774;0.67050179756341044;-0.073816424486715937;0.57556393843195341;-0.51965569737353523;-0.18188984516686479;0.86607142217565303;0.73125255890540142;-0.64495249089610818;-0.93647428229135443;-0.40009041011534546]
      mask Display: e = 0.06;c1 = [120 150 230]/255;c2 = ([120 150 230]+0)/383;c3 = ([120 150 230]+128)/383;patch([0 1 1 0],[0 0 1 1],c1);patch([0 1 1 1-e 1-e 0+e],[0 0 1 1-e 0+e 0+e],c2);patch([0 0 1 1-e 0+e 0+e],[0 1 1 1-e 1-e 0+e],c3);plot([0 1 1 0 0],[0 0 1 1 0]);disp('weights');
  "IW{2,1}(8,:)'" : Constant  Value=[-0.30553229113642855;-0.86617970816336753;0.80966053392488124;0.73667050983796711;0.55823784497271101;-0.33590280249045451;-0.60451247500270233;-0.58209177199353956;1.0210052919903716;0.84444810197350606;0.52856340224068843;-0.98749391120638275;-0.0056472306723189718;-0.10540987827334283;-0.87512766987745338;-0.11142913536062568;0.71518295146263799;-0.43139353749721426;0.072385775284947634;0.15863729940722318;-0.55777468924654894;-0.88679865313365092;0.8911238162212477;0.90535078022499804;-0.10090852099170307]
      mask Display: e = 0.06;c1 = [120 150 230]/255;c2 = ([120 150 230]+0)/383;c3 = ([120 150 230]+128)/383;patch([0 1 1 0],[0 0 1 1],c1);patch([0 1 1 1-e 1-e 0+e],[0 0 1 1-e 0+e 0+e],c2);patch([0 0 1 1-e 0+e 0+e],[0 1 1 1-e 1-e 0+e],c3);plot([0 1 1 0 0],[0 0 1 1 0]);disp('weights');
  "IW{2,1}(9,:)'" : Constant  Value=[-0.84684298995683449;-0.37019591551771869;-0.55376976280087664;0.12344265495216562;-0.84923893207729106;0.16568695710108308;-0.76438244086725848;0.69900075451372412;0.42721309150794701;-0.088375532145569771;-0.88749011741605355;0.59389251938969478;-0.69364985314987204;0.9602263394930024;-0.72711075038090944;-1.2273127636818846;-0.92336463147851044;0.26447236942855418;0.54219428867148756;-0.2032508086272545;-1.0041647679335237;0.002462606844041986;0.035273874045691607;0.6246092862271253;-0.3671125044658462]
      mask Display: e = 0.06;c1 = [120 150 230]/255;c2 = ([120 150 230]+0)/383;c3 = ([120 150 230]+128)/383;patch([0 1 1 0],[0 0 1 1],c1);patch([0 1 1 1-e 1-e 0+e],[0 0 1 1-e 0+e 0+e],c2);patch([0 0 1 1-e 0+e 0+e],[0 1 1 1-e 1-e 0+e],c3);plot([0 1 1 0 0],[0 0 1 1 0]);disp('weights');
  Mux : Mux  Inputs=40
      mask Display: e = 0.06;c1 = [120 150 230]/255;c2 = ([120 150 230]+0)/383;c3 = ([120 150 230]+128)/383;patch([0 1 1 0],[0 0 1 1],c1);patch([0 1 1 1-e 1-e 0+e],[0 0 1 1-e 0+e 0+e],c2);patch([0 0 1 1-e 0+e 0+e],[0 1 1 1-e 1-e 0+e],c3);plot([0 1 1 0 0],[0 0 1 1 0]);disp('Mux');
  dotprod{1..40} (40 alike) : neural/Weight Functions/dotprod  SystemSampleTime=-1
  "lz{2,1}" : Outport
      mask Display: e = 0.06;c1 = [120 230 180]/255;c2 = ([120 230 180]+0)/(256+128);c3 = ([120 230 180]+128)/(256+128);patch([0 1 1 0],[0 0 1 1],c1);patch([0 1 1 1-e 1-e 0+e],[0 0 1 1-e 0+e 0+e],c2);patch([0 0 1 1-e 0+e 0+e],[0 1 1 1-e 1-e 0+e],c3);plot([0 1 1 0 0],[0 0 1 1 0]);
  wires:
  "IW{2,1}(1,:)'"/1 -> dotprod1/1
  "ad{2,1}"/1 -> dotprod1/2, dotprod2/2, dotprod3/2, dotprod4/2, dotprod5/2, dotprod6/2, dotprod7/2, dotprod8/2, dotprod9/2, dotprod10/2, dotprod11/2, dotprod12/2, dotprod13/2, dotprod14/2, dotprod15/2, dotprod16/2, dotprod17/2, dotprod18/2, dotprod19/2, dotprod20/2, dotprod21/2, dotprod22/2, dotprod23/2, dotprod24/2, dotprod25/2, dotprod26/2, dotprod27/2, dotprod28/2, dotprod29/2, dotprod30/2, dotprod31/2, dotprod32/2, dotprod33/2, dotprod34/2, dotprod35/2, dotprod36/2, dotprod37/2, dotprod38/2, dotprod39/2, dotprod40/2
  dotprod1/1 -> Mux/1
  "IW{2,1}(2,:)'"/1 -> dotprod2/1
  dotprod2/1 -> Mux/2
  "IW{2,1}(3,:)'"/1 -> dotprod3/1
  dotprod3/1 -> Mux/3
  "IW{2,1}(4,:)'"/1 -> dotprod4/1
  dotprod4/1 -> Mux/4
  "IW{2,1}(5,:)'"/1 -> dotprod5/1
  dotprod5/1 -> Mux/5
  "IW{2,1}(6,:)'"/1 -> dotprod6/1
  dotprod6/1 -> Mux/6
  "IW{2,1}(7,:)'"/1 -> dotprod7/1
  dotprod7/1 -> Mux/7
  "IW{2,1}(8,:)'"/1 -> dotprod8/1
  dotprod8/1 -> Mux/8
  "IW{2,1}(9,:)'"/1 -> dotprod9/1
  dotprod9/1 -> Mux/9
  "IW{2,1}(10,:)'"/1 -> dotprod10/1
  dotprod10/1 -> Mux/10
  "IW{2,1}(11,:)'"/1 -> dotprod11/1
  dotprod11/1 -> Mux/11
  "IW{2,1}(12,:)'"/1 -> dotprod12/1
  dotprod12/1 -> Mux/12
  "IW{2,1}(13,:)'"/1 -> dotprod13/1
  dotprod13/1 -> Mux/13
  "IW{2,1}(14,:)'"/1 -> dotprod14/1
  dotprod14/1 -> Mux/14
  "IW{2,1}(15,:)'"/1 -> dotprod15/1
  dotprod15/1 -> Mux/15
  "IW{2,1}(16,:)'"/1 -> dotprod16/1
  dotprod16/1 -> Mux/16
  "IW{2,1}(17,:)'"/1 -> dotprod17/1
  dotprod17/1 -> Mux/17
  "IW{2,1}(18,:)'"/1 -> dotprod18/1
  dotprod18/1 -> Mux/18
  "IW{2,1}(19,:)'"/1 -> dotprod19/1
  dotprod19/1 -> Mux/19
  "IW{2,1}(20,:)'"/1 -> dotprod20/1
  dotprod20/1 -> Mux/20
  "IW{2,1}(21,:)'"/1 -> dotprod21/1
  dotprod21/1 -> Mux/21
  "IW{2,1}(22,:)'"/1 -> dotprod22/1
  dotprod22/1 -> Mux/22
  "IW{2,1}(23,:)'"/1 -> dotprod23/1
  dotprod23/1 -> Mux/23
  "IW{2,1}(24,:)'"/1 -> dotprod24/1
  dotprod24/1 -> Mux/24
  "IW{2,1}(25,:)'"/1 -> dotprod25/1
  dotprod25/1 -> Mux/25
  "IW{2,1}(26,:)'"/1 -> dotprod26/1
  dotprod26/1 -> Mux/26
  "IW{2,1}(27,:)'"/1 -> dotprod27/1
  dotprod27/1 -> Mux/27
  "IW{2,1}(28,:)'"/1 -> dotprod28/1
  dotprod28/1 -> Mux/28
  "IW{2,1}(29,:)'"/1 -> dotprod29/1
  dotprod29/1 -> Mux/29
  "IW{2,1}(30,:)'"/1 -> dotprod30/1
  dotprod30/1 -> Mux/30
  "IW{2,1}(31,:)'"/1 -> dotprod31/1
  dotprod31/1 -> Mux/31
  "IW{2,1}(32,:)'"/1 -> dotprod32/1
  dotprod32/1 -> Mux/32
  "IW{2,1}(33,:)'"/1 -> dotprod33/1
  dotprod33/1 -> Mux/33
  "IW{2,1}(34,:)'"/1 -> dotprod34/1
  dotprod34/1 -> Mux/34
  "IW{2,1}(35,:)'"/1 -> dotprod35/1
  dotprod35/1 -> Mux/35
  "IW{2,1}(36,:)'"/1 -> dotprod36/1
  dotprod36/1 -> Mux/36
  "IW{2,1}(37,:)'"/1 -> dotprod37/1
  dotprod37/1 -> Mux/37
  "IW{2,1}(38,:)'"/1 -> dotprod38/1
  dotprod38/1 -> Mux/38
  "IW{2,1}(39,:)'"/1 -> dotprod39/1
  dotprod39/1 -> Mux/39
  "IW{2,1}(40,:)'"/1 -> dotprod40/1
  dotprod40/1 -> Mux/40
  Mux/1 -> "lz{2,1}"/1

== system MLP_networks/net_loc_rod_8_9/Layer 3/Delays 1 ==
  "p{3}" : Inport  PortDimensions=40
      mask Display: e = 0.06;c1 = [120 230 180]/255;c2 = ([120 230 180]+0)/(256+128);c3 = ([120 230 180]+128)/(256+128);patch([0 1 1 0],[0 0 1 1],c1);patch([0 1 1 1-e 1-e 0+e],[0 0 1 1-e 0+e 0+e],c2);patch([0 0 1 1-e 0+e 0+e],[0 1 1 1-e 1-e 0+e],c3);plot([0 1 1 0 0],[0 0 1 1 0]);
  mux : Mux  Inputs=1
      mask Display: e = 0.06;c1 = [120 150 230]/255;c2 = ([120 150 230]+0)/383;c3 = ([120 150 230]+128)/383;patch([0 1 1 0],[0 0 1 1],c1);patch([0 1 1 1-e 1-e 0+e],[0 0 1 1-e 0+e 0+e],c2);patch([0 0 1 1-e 0+e 0+e],[0 1 1 1-e 1-e 0+e],c3);plot([0 1 1 0 0],[0 0 1 1 0]);disp('Mux')
  "pd{3,2}" : Outport
      mask Display: e = 0.06;c1 = [120 230 180]/255;c2 = ([120 230 180]+0)/(256+128);c3 = ([120 230 180]+128)/(256+128);patch([0 1 1 0],[0 0 1 1],c1);patch([0 1 1 1-e 1-e 0+e],[0 0 1 1-e 0+e 0+e],c2);patch([0 0 1 1-e 0+e 0+e],[0 1 1 1-e 1-e 0+e],c3);plot([0 1 1 0 0],[0 0 1 1 0]);
  wires:
  "p{3}"/1 -> mux/1
  mux/1 -> "pd{3,2}"/1

== system MLP_networks/net_loc_rod_8_9/Layer 3/LW{3,2} ==
  "ad{3,2}" : Inport  PortDimensions=40
      mask Display: e = 0.06;c1 = [120 230 180]/255;c2 = ([120 230 180]+0)/(256+128);c3 = ([120 230 180]+128)/(256+128);patch([0 1 1 0],[0 0 1 1],c1);patch([0 1 1 1-e 1-e 0+e],[0 0 1 1-e 0+e 0+e],c2);patch([0 0 1 1-e 0+e 0+e],[0 1 1 1-e 1-e 0+e],c3);plot([0 1 1 0 0],[0 0 1 1 0]);
  "IW{3,2}(1,:)'" : Constant  Value=[0.32376944664437463;1.0671260685907464;0.086615085919476087;0.45711678721492455;-0.88639209752428594;-0.85756531218717358;-0.57809808272177798;0.5858839479296678;0.57987760709210678;0.65360473887572557;-0.35994050166718328;-1.0228857127537725;-0.19587289604082067;-0.77369993139411963;-0.56904142757082354;-0.72012333590135702;0.0043076560260231185;0.56819175014574697;0.4305725803897032;0.93778237759050787;-0.30381005871498123;0.82777509187326581;0.37837873903712549;0.42570911150749613;-0.51571870454573387;0.84385791604438953;-0.53520056486716705;0.1212095007337415;0.16423369192451126;0.77826762235172164;0.38821292529394053;-1.0025845993086693;-0.29961877482603683;-0.53750988206769545;-0.69567554814672461;-0.7961736002161125;-0.7235605550502977;0.48502478419908152;0.92522107335399462;1.1601792249495149]
      mask Display: e = 0.06;c1 = [120 150 230]/255;c2 = ([120 150 230]+0)/383;c3 = ([120 150 230]+128)/383;patch([0 1 1 0],[0 0 1 1],c1);patch([0 1 1 1-e 1-e 0+e],[0 0 1 1-e 0+e 0+e],c2);patch([0 0 1 1-e 0+e 0+e],[0 1 1 1-e 1-e 0+e],c3);plot([0 1 1 0 0],[0 0 1 1 0]);disp('weights');
  Mux : Mux  Inputs=1
      mask Display: e = 0.06;c1 = [120 150 230]/255;c2 = ([120 150 230]+0)/383;c3 = ([120 150 230]+128)/383;patch([0 1 1 0],[0 0 1 1],c1);patch([0 1 1 1-e 1-e 0+e],[0 0 1 1-e 0+e 0+e],c2);patch([0 0 1 1-e 0+e 0+e],[0 1 1 1-e 1-e 0+e],c3);plot([0 1 1 0 0],[0 0 1 1 0]);disp('Mux');
  dotprod1 : neural/Weight Functions/dotprod  SystemSampleTime=-1
  "lz{3,2}" : Outport
      mask Display: e = 0.06;c1 = [120 230 180]/255;c2 = ([120 230 180]+0)/(256+128);c3 = ([120 230 180]+128)/(256+128);patch([0 1 1 0],[0 0 1 1],c1);patch([0 1 1 1-e 1-e 0+e],[0 0 1 1-e 0+e 0+e],c2);patch([0 0 1 1-e 0+e 0+e],[0 1 1 1-e 1-e 0+e],c3);plot([0 1 1 0 0],[0 0 1 1 0]);
  wires:
  "IW{3,2}(1,:)'"/1 -> dotprod1/1
  "ad{3,2}"/1 -> dotprod1/2
  dotprod1/1 -> Mux/1
  Mux/1 -> "lz{3,2}"/1
